simulink library "Lib_ReferencePointCalculation"  (R2019b)
settings: Solver=VariableStepAuto  StartTime=0.0  StopTime=10.0  RelTol=1e-3
undefined symbols (not defined in the file): trajectory_timeshift_speed_threshold
settings Model: Creator=esterle  LastModifiedBy=kessler
settings DataIOCC: ReturnWorkspaceOutputs=off
settings DebuggingCC: ArithmeticOperatorsInVariantConditions=warning
settings SFSimCC: SimUseLocalCustomCode=off  CustomCodeUndefinedFunction=UseInterfaceOnly
settings RTWCC: RTWUseLocalCustomCode=off

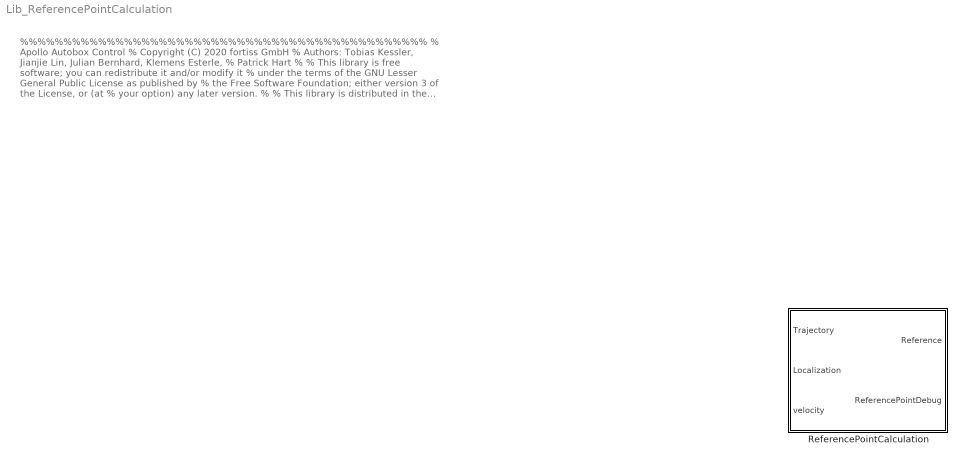
== system Lib_ReferencePointCalculation ==
  note: %%%%%%%%%%%%%%%%%%%%%%%%%%%%%%%%%%%%%%%%%%%%%%%
      | % Apollo Autobox Control
      | % Copyright (C) 2020 fortiss GmbH
      | % Authors: Tobias Kessler, Jianjie Lin, Julian Bernhard, Klemens Esterle,
      | % Patrick Hart
      | %
      | % This library is free software; you can redistribute it and/or modify it
      | % under the terms of the GNU Lesser General Public License as published by
      | % the Free Software Foundation; either version 3 of the License, or (at
      | % your option) any later version.
      | %
      | % This library is distributed in the hope that it will be useful, but
      | % WITHOUT ANY WARRANTY; without even the implied warranty of
      | % MERCHANTABILITY or FITNESS FOR A PARTICULAR PURPOSE. See the GNU Lesser
      | % General Public License for more details.
      | %
      | % You should have received a copy of the GNU Lesser General Public License
      | % along with this library; if not, write to the Free Software Foundation,
      | % Inc., 51 Franklin Street, Fifth Floor, Boston, MA 02110-1301, USA.
      | %%%%%%%%%%%%%%%%%%%%%%%%%%%%%%%%%%%%%%%%%%%%%%%
  ReferencePointCalculation : Subsystem

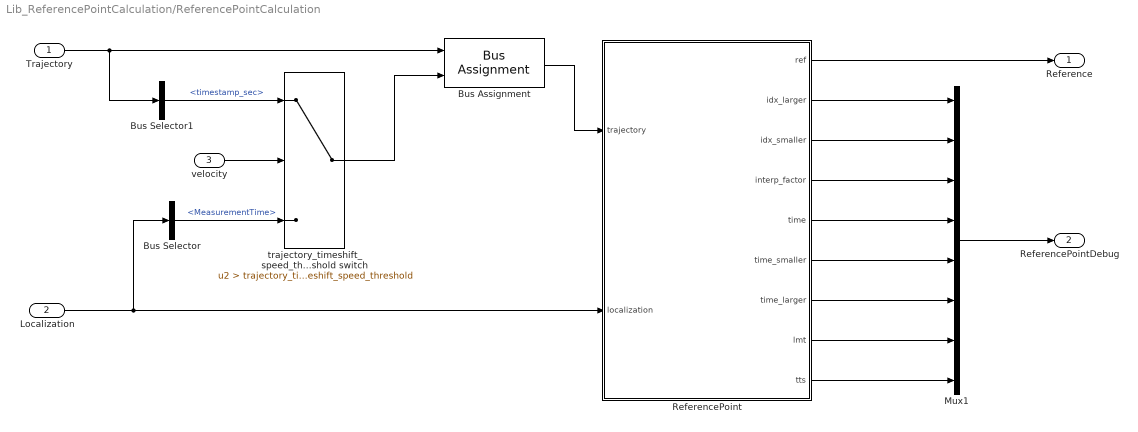
== system Lib_ReferencePointCalculation/ReferencePointCalculation ==
  Trajectory : Inport  OutDataTypeStr=Bus: ControlTrajectory  BusOutputAsStruct=on
  Localization : Inport  Port=2  OutDataTypeStr=Bus: LocalizationToAutobox  BusOutputAsStruct=on
  velocity : Inport  Port=3
  Bus Assignment : BusAssignment  AssignedSignals=timestamp_sec
  Bus Selector : BusSelector  OutputSignals=MeasurementTime
  Bus Selector1 : BusSelector  OutputSignals=timestamp_sec
  Mux1 : Mux  Inputs=8
  ReferencePoint : MATLAB Function  TreatAsAtomicUnit=on
  trajectory_timeshift_speed_threshold switch : Switch  Criteria=u2 > Threshold  Threshold=trajectory_timeshift_speed_threshold
  Reference : Outport  VectorParamsAs1DForOutWhenUnconnected=off
  ReferencePointDebug : Outport  Port=2  VectorParamsAs1DForOutWhenUnconnected=off
  wires:
  Bus Assignment/1 -> ReferencePoint/1(trajectory)
  Bus Selector/1 -> trajectory_timeshift_speed_threshold switch/3  "<MeasurementTime>"
  Bus Selector1/1 -> trajectory_timeshift_speed_threshold switch/1  "<timestamp_sec>"
  trajectory_timeshift_speed_threshold switch/1 -> Bus Assignment/2
  velocity/1 -> trajectory_timeshift_speed_threshold switch/2
  ReferencePoint/9(tts) -> Mux1/8
  ReferencePoint/8(lmt) -> Mux1/7
  ReferencePoint/6(time_smaller) -> Mux1/5
  ReferencePoint/7(time_larger) -> Mux1/6
  ReferencePoint/5(time) -> Mux1/4
  Mux1/1 -> ReferencePointDebug/1
  ReferencePoint/4(interp_factor) -> Mux1/3
  ReferencePoint/3(idx_smaller) -> Mux1/2
  ReferencePoint/2(idx_larger) -> Mux1/1
  Trajectory/1 -> Bus Selector1/1, Bus Assignment/1
  Localization/1 -> ReferencePoint/2(localization), Bus Selector/1
  ReferencePoint/1(ref) -> Reference/1

== matlab function Lib_ReferencePointCalculation/ReferencePointCalculation/ReferencePoint ==
  data: trajectory input; localization input Bus: LocalizationToAutobox; ref output Bus: TrajectoryPoint; idx_larger output double; idx_smaller output double; interp_factor output; time output; time_smaller output; time_larger output; lmt output; tts output
function [ref, idx_larger, idx_smaller, interp_factor, time, time_smaller, time_larger, lmt, tts] = ref_point_determination(trajectory, localization)

[ref, idx_larger, idx_smaller, interp_factor, time, time_smaller, time_larger, lmt, tts] = ref_point_determination_time_based(trajectory, localization);
